simulink library "lib"  (R2018a)
settings: Solver=VariableStepAuto  StartTime=0.0  StopTime=10.0  RelTol=1e-3
settings Model: Creator=Toni  LastModifiedBy=Toni

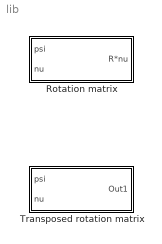
== system lib ==
  Rotation matrix : Subsystem
  Transposed rotation matrix : Subsystem

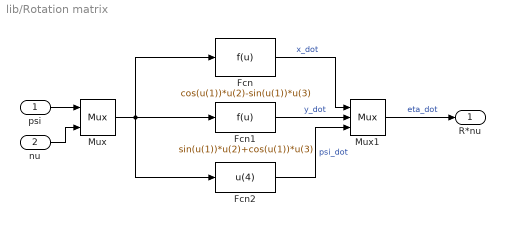
== system lib/Rotation matrix ==
  psi : Inport
  nu : Inport  Port=2
  Fcn : Fcn  Expr=cos(u(1))*u(2)-sin(u(1))*u(3)
  Fcn1 : Fcn  Expr=sin(u(1))*u(2)+cos(u(1))*u(3)
  Fcn2 : Fcn  Expr=u(4)
  Mux : Mux  Inputs=2
  Mux1 : Mux  Inputs=3
  R*nu : Outport
  wires:
  Fcn1/1 -> Mux1/2  "y_dot"
  Mux/1 -> Fcn2/1, Fcn1/1, Fcn/1
  psi/1 -> Mux/1
  Mux1/1 -> R*nu/1  "eta_dot"
  Fcn/1 -> Mux1/1  "x_dot"
  Fcn2/1 -> Mux1/3  "psi_dot"
  nu/1 -> Mux/2

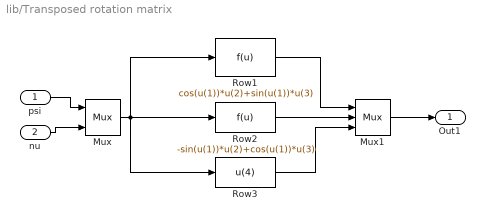
== system lib/Transposed rotation matrix ==
  psi : Inport
  nu : Inport  Port=2
  Mux : Mux  Inputs=2
  Mux1 : Mux  Inputs=3
  Row1 : Fcn  Expr=cos(u(1))*u(2)+sin(u(1))*u(3)
  Row2 : Fcn  Expr=-sin(u(1))*u(2)+cos(u(1))*u(3)
  Row3 : Fcn  Expr=u(4)
  Out1 : Outport
  wires:
  Mux/1 -> Row1/1, Row2/1, Row3/1
  Row1/1 -> Mux1/1
  psi/1 -> Mux/1
  nu/1 -> Mux/2
  Row2/1 -> Mux1/2
  Mux1/1 -> Out1/1
  Row3/1 -> Mux1/3
